simulink model "Control_Bluetooth"  (R2024b)
settings: Solver=FixedStepDiscrete  StartTime=0.0  StopTime=inf  FixedStep=0.01  RelTol=1e-3  EnableMultiTasking=on
settings Model: ExtModeTrigDuration=2  Creator=Chenfu  LastModifiedBy=Chenfu
settings SolverCC: AutoInsertRateTranBlk=on
settings OptimizationCC: DefaultParameterBehavior=Inlined  EnhancedBackFolding=on  PassReuseOutputArgsAs=Individual arguments  ZeroExternalMemoryAtStartup=off  ZeroInternalMemoryAtStartup=off  MaxStackSize=64  OptimizeBlockOrder=speed  DifferentSizesBufferReuse=on  OptimizationCustomize=off  EfficientTunableParamExpr=on
settings DebuggingCC: ParameterTunabilityLossMsg=error
settings HardwareCC: ProdBitPerInt=16  ProdBitPerPointer=16  ProdBitPerSizeT=16  ProdBitPerPtrDiffT=16  ProdLargestAtomicFloat=None  ProdWordSize=8  ProdHWDeviceType=Atmel->AVR  UseEmbeddedCoderFeatures=off  UseSimulinkCoderFeatures=off
settings SFSimCC: MATLABDynamicMemAlloc=off
settings RTWCC: Description=Embedded Coder  SystemTargetFile=ert.tlc  HardwareBoard=Arduino Mega 2560  TemplateMakefile=ert_default_tmf  Toolchain=Arduino AVR  BuildConfiguration=Faster Runs  GPUComputeCapability=3.5
settings CodeAppCC: ForceParamTrailComments=on  IgnoreCustomStorageClasses=off  OperatorAnnotations=on  SimulinkDataObjDesc=on  SFDataObjDesc=on  InsertBlockDesc=on
settings ERTTargetCC: SupportContinuousTime=on  SupportNonInlinedSFcns=on  SupportVariableSizeSignals=on  ExtModeTransport=3  ExtModeStaticAlloc=on  ExtModeAutomaticAllocSize=off  ExtModeStaticAllocSize=2048  ExtModeMexFile=ext_xcp  ExtModeIntrfLevel=Level2 - Open

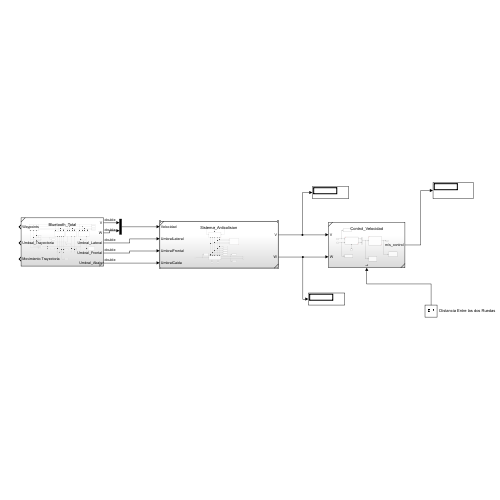
[thumbnail: Simulink's stored preview of the top-level diagram]
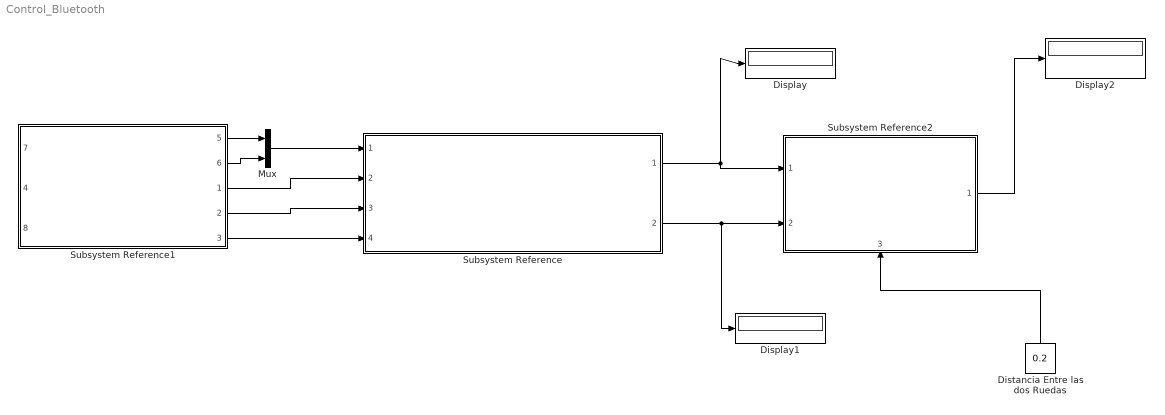
== system Control_Bluetooth ==
  Display : Display
  Display1 : Display
  Display2 : Display
  Distancia Entre las dos Ruedas : Constant  Value=0.2
  Mux : Mux  Inputs=2
  Subsystem Reference : Subsystem  ReferencedSubsystem=Sistema_Anticolision
  Subsystem Reference1 : Subsystem  ReferencedSubsystem=Bluetooth_Total
      settings: PortSchema="{\"entries\":[{\"content\":{\"sides\":[{\"content\":{\"connectorIds\":[\"Out7\",\"Out4\",\"Out8\"]},\"type\":\"ConnectorPlacement.EquallySpacedRectSide\",\"uuid\":\"e546e10f-6993-4aa1-adbd-c05ce222087d\"},{\"content\":{\"connectorIds\":[\"Out5\",\"Out6\",\"Out1\",\"Out2\",\"Out3\"],\"side\":\"RIGHT\"},\"type\":\"ConnectorPlacement.EquallySpacedRectSide\",\"uuid\":\"c6902324-8bb8-49b8-9b1e-f6c09f9f2113\"},{\"content\":{\"side\":\"TOP\"},\"type\":\"ConnectorPlacement.EquallySpacedRectSide\",\"uuid\":\"da8c9621-de83-4872-91e8-7b7438518584\"}]},\"type\":\"ConnectorPlacement.EquallySpacedConnector\",\"uuid\":\"5840c5b0-eeea-4fcc-b8e1-1389fac507e0\"}],\"packageUris\":[\"http://schema.mathworks.com/mf0/Connector/R2020b\"],\"version\":\"1.0\"}"
  Subsystem Reference2 : Subsystem  ReferencedSubsystem=Control_Velocidad
      settings: PortSchema="{\"entries\":[{\"content\":{\"sides\":[{\"content\":{\"connectorIds\":[\"In1\",\"In2\"]},\"type\":\"ConnectorPlacement.EquallySpacedRectSide\",\"uuid\":\"296ec3ce-a2cd-47ea-b6d2-93e60c3d408c\"},{\"content\":{\"connectorIds\":[\"Out1\"],\"side\":\"RIGHT\"},\"type\":\"ConnectorPlacement.EquallySpacedRectSide\",\"uuid\":\"4b69a479-ec69-4494-a3b5-f93cec5223a5\"},{\"content\":{\"side\":\"TOP\"},\"type\":\"ConnectorPlacement.EquallySpacedRectSide\",\"uuid\":\"61ce2b34-b784-4c5c-9397-e479630368ea\"},{\"content\":{\"connectorIds\":[\"In3\"],\"side\":\"BOTTOM\"},\"type\":\"ConnectorPlacement.EquallySpacedRectSide\",\"uuid\":\"d41f115b-0f7b-4d66-895a-77e45f9c625f\"}]},\"type\":\"ConnectorPlacement.EquallySpacedConnector\",\"uuid\":\"e1451c87-18e2-4848-a5d0-d80c1278d298\"}],\"packageUris\":[\"http://schema.mathworks.com/mf0/Connector/R2020b\"],\"version\":\"1.0\"}"
  wires:
  Subsystem Reference2/1 -> Display2/1
  Subsystem Reference/1 -> Display/1, Subsystem Reference2/1
  Subsystem Reference/2 -> Display1/1, Subsystem Reference2/2
  Distancia Entre las dos Ruedas/1 -> Subsystem Reference2/3
  Subsystem Reference1/5 -> Mux/1
  Subsystem Reference1/6 -> Mux/2
  Mux/1 -> Subsystem Reference/1
  Subsystem Reference1/1 -> Subsystem Reference/2
  Subsystem Reference1/2 -> Subsystem Reference/3
  Subsystem Reference1/3 -> Subsystem Reference/4
